simulink model "DCAC"  (R2023b)
settings: Solver=FixedStepDiscrete  StartTime=0.0  StopTime=5  FixedStep=SIM_Ts  RelTol=1e-3
PreLoadFcn:
  | addpath("Sim\");
  | run(Sim_PreLoad_DCAC.mlx);
undefined symbols (not defined in the file): C, f_Vref, L, R_Load, SIM_Ts, t_Vref, Ts, V_DC
libraries: spsSeriesRLCBranchLib x19, spsMosfetLib x12, simulink x10, spsVoltageMeasurementLib x9, spsOnDelayLib x8, spsDCVoltageSourceLib x1, spsGroundLib x1, spsMultimeterLib x1, spspowerguiLib x1
settings Model: Creator=VanillaC  LastModifiedBy=VanillaC
settings DataIOCC: ReturnWorkspaceOutputs=off
settings OptimizationCC: DefaultParameterBehavior=Inlined  EnhancedBackFolding=on  PassReuseOutputArgsAs=Individual arguments  ZeroExternalMemoryAtStartup=off  ZeroInternalMemoryAtStartup=off  OptimizeBlockOrder=speed  DifferentSizesBufferReuse=on  OptimizationCustomize=off  EfficientTunableParamExpr=on
settings DebuggingCC: ParameterTunabilityLossMsg=error
settings SFSimCC: MATLABDynamicMemAlloc=off
settings RTWCC: Description=Embedded Coder  SystemTargetFile=ert.tlc  GenCodeOnly=on  TemplateMakefile=ert_default_tmf
settings CodeAppCC: ForceParamTrailComments=on  IgnoreCustomStorageClasses=off  OperatorAnnotations=on  SimulinkDataObjDesc=on  SFDataObjDesc=on  InsertBlockDesc=on  MATLABSourceComments=on
settings ERTTargetCC: TargetLangStandard=C99 (ISO)  GenerateSampleERTMain=on  SupportContinuousTime=on  InlinedParameterPlacement=NonHierarchical  ERTCustomFileTemplate=example_file_process.tlc

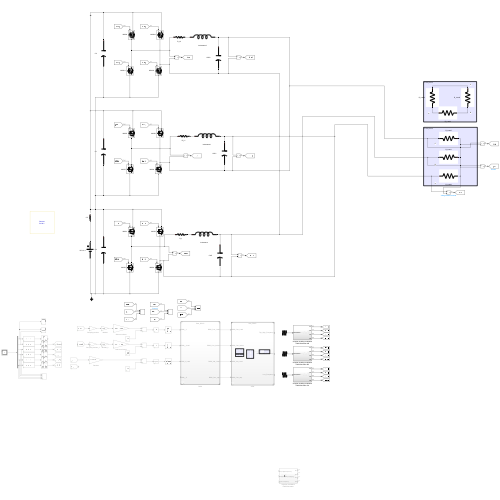
[thumbnail: Simulink's stored preview of the top-level diagram]
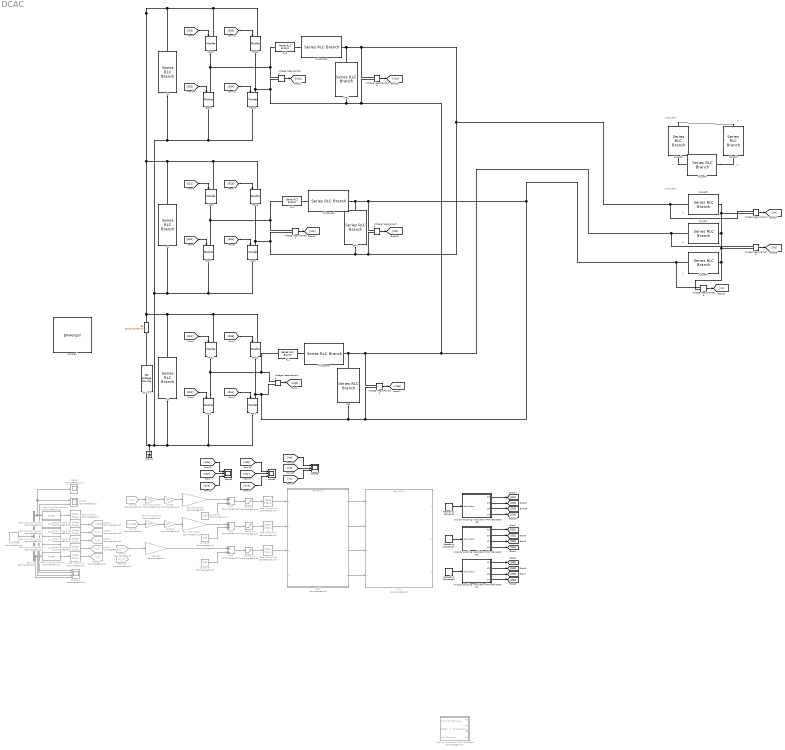
== system DCAC ==
  note: A
  note: Subsystem
  note: B
  note: C
  note: A
  note: Subsystem
  note: C
  note: B
  ASW : ModelReference  Commented=on  ModelNameDialog=Asw_DCAC.slx  SimulationMode=Normal  ModelReferenceVersion=7.2
  Add3 : Sum  Commented=on
  Add4 : Sum  Commented=on
  Add5 : Sum  Commented=on
  BSW : ModelReference  Commented=on  ModelNameDialog=Bsw_DCAC.slx  SimulationMode=Normal  ModelReferenceVersion=1.11
      settings: PortSchema="{\"entries\":[{\"content\":{\"sides\":[{\"content\":{\"connectorIds\":[\"In2\",\"In1\",\"In3\",\"In4\"]},\"type\":\"ConnectorPlacement.EquallySpacedRectSide\",\"uuid\":\"b2b7a57c-7cf1-4c06-9e54-7dc01d62324f\"},{\"content\":{\"connectorIds\":[\"Out1\",\"Out2\",\"Out3\",\"Out4\"],\"side\":\"RIGHT\"},\"type\":\"ConnectorPlacement.EquallySpacedRectSide\",\"uuid\":\"58967db2-deee-4275-8865-8f1f6f5d01b9\"},{\"content\":{\"side\":\"TOP\"},\"type\":\"ConnectorPlacement.EquallySpacedRectSide\",\"uuid\":\"d9088037-5ecd-44ee-9dae-30c0aa6e59e3\"}]},\"type\":\"ConnectorPlacement.EquallySpacedConnector\",\"uuid\":\"be37a7a2-a861-4ca5-b50a-1f8ecf43409b\"}],\"packageUris\":[\"http://schema.mathworks.com/mf0/Connector/R2020b\"],\"version\":\"1.0\"}"
  C1 : spsSeriesRLCBranchLib/Series RLC Branch  LConnTagsString=__new0  RConnTagsString=__new0  BranchType=C  Resistance=1e-9  Inductance=1e-3  SetiL0=off  InitialCurrent=0  Capacitance=2.2e3  Setx0=off  InitialVoltage=0  Measurements=None
  C2 : spsSeriesRLCBranchLib/Series RLC Branch  LConnTagsString=__new0  RConnTagsString=__new0  BranchType=C  Resistance=1e-9  Inductance=1e-3  SetiL0=off  InitialCurrent=0  Capacitance=2.2e3  Setx0=off  InitialVoltage=0  Measurements=None
  C3 : spsSeriesRLCBranchLib/Series RLC Branch  LConnTagsString=__new0  RConnTagsString=__new0  BranchType=C  Resistance=1e-9  Inductance=1e-3  SetiL0=off  InitialCurrent=0  Capacitance=2.2e3  Setx0=off  InitialVoltage=0  Measurements=None
  C5 : spsSeriesRLCBranchLib/Series RLC Branch  LConnTagsString=__new0  RConnTagsString=__new0  BranchType=R  Resistance=1e-10  Inductance=1e-3  SetiL0=off  InitialCurrent=0  Capacitance=2.2e-3  Setx0=off  InitialVoltage=0  Measurements=None
  CAP : spsSeriesRLCBranchLib/Series RLC Branch  LConnTagsString=__new0  RConnTagsString=__new0  BranchType=C  Resistance=1000  Inductance=1e-3  SetiL0=off  InitialCurrent=0  Capacitance=C  Setx0=off  InitialVoltage=0  Measurements=Branch voltage and current
  CAP1 : spsSeriesRLCBranchLib/Series RLC Branch  LConnTagsString=__new0  RConnTagsString=__new0  BranchType=C  Resistance=1000  Inductance=1e-3  SetiL0=off  InitialCurrent=0  Capacitance=C  Setx0=off  InitialVoltage=0  Measurements=Branch voltage and current
  CAP2 : spsSeriesRLCBranchLib/Series RLC Branch  LConnTagsString=__new0  RConnTagsString=__new0  BranchType=C  Resistance=1000  Inductance=1e-3  SetiL0=off  InitialCurrent=0  Capacitance=C  Setx0=off  InitialVoltage=0  Measurements=Branch voltage and current
  Constant3 : Constant  Commented=on  Value=1.65  OutDataTypeStr=single  SampleTime=-1
  Constant4 : Constant  Commented=on  Value=1.65  OutDataTypeStr=single  SampleTime=-1
  Constant5 : Constant  Commented=on  Value=1.65  OutDataTypeStr=single  SampleTime=-1
  DC Vin 1 : spsDCVoltageSourceLib/DC Voltage Source  Amplitude=V_DC  Measurements=None
  Data Type Conversion{1..6} (6 alike) : DataTypeConversion  Commented=on  OutDataTypeStr=single  SaturateOnIntegerOverflow=off  RndMeth=Floor
  Demux1 : Demux  Commented=on  Outputs=6
  From16 : From  Commented=on  GotoTag=U_C
  From19 : From  Commented=on  GotoTag=I_Load
  From20 : From  Commented=on  GotoTag=I_L
  From21 : From  Commented=on  GotoTag=U_Load
  Gain error factor : Gain  Commented=on  Gain=3000/(10+3000)
  Gain error factor1 : Gain  Commented=on  Gain=3000/(10+3000)
  Goto19 : Goto  Commented=on  GotoTag=I_Load
  Goto20 : Goto  Commented=on  GotoTag=U_L
  Goto21 : Goto  Commented=on  GotoTag=I_L
  Goto22 : Goto  Commented=on  GotoTag=U_C
  Goto23 : Goto  Commented=on  GotoTag=I_C
  Ground : spsGroundLib/Ground  LConnTagsString=a
  INA296 : Gain  Commented=on  Gain=100
  INA296_2 : Gain  Commented=on  Gain=100
  Inductance : spsSeriesRLCBranchLib/Series RLC Branch  LConnTagsString=__new0  RConnTagsString=__new0  BranchType=L  Resistance=0.005  Inductance=L  SetiL0=off  InitialCurrent=0  Capacitance=470e-6  Setx0=off  InitialVoltage=0  Measurements=Branch voltage and current
  Inductance1 : spsSeriesRLCBranchLib/Series RLC Branch  LConnTagsString=__new0  RConnTagsString=__new0  BranchType=L  Resistance=0.005  Inductance=L  SetiL0=off  InitialCurrent=0  Capacitance=470e-6  Setx0=off  InitialVoltage=0  Measurements=Branch voltage and current
  Inductance2 : spsSeriesRLCBranchLib/Series RLC Branch  LConnTagsString=__new0  RConnTagsString=__new0  BranchType=L  Resistance=0.005  Inductance=L  SetiL0=off  InitialCurrent=0  Capacitance=470e-6  Setx0=off  InitialVoltage=0  Measurements=Branch voltage and current
  MOS{1..12} (12 alike) : spsMosfetLib/Mosfet  Ron=1e-9  Lon=0  Rd=1e-9  Vfd=0.7  IC=0  Rs=1e5  Cs=inf  Measurements=off
  Multimeter : spsMultimeterLib/Multimeter  Commented=on  L=8  sel=[4 8 2 6 1 5]  yselected={}  Gain=[1 1 1 1 1 1]  OutputType=Complex  PlotAtSimulationStop=off  PhasorSimulation=off
  R_L : spsSeriesRLCBranchLib/Series RLC Branch  LConnTagsString=__new0  RConnTagsString=__new0  BranchType=R  Resistance=1e-10  Inductance=1e-3  SetiL0=off  InitialCurrent=0  Capacitance=470e-6  Setx0=off  InitialVoltage=0  Measurements=None
  R_L1 : spsSeriesRLCBranchLib/Series RLC Branch  LConnTagsString=__new0  RConnTagsString=__new0  BranchType=R  Resistance=1e-10  Inductance=1e-3  SetiL0=off  InitialCurrent=0  Capacitance=470e-6  Setx0=off  InitialVoltage=0  Measurements=None
  R_L2 : spsSeriesRLCBranchLib/Series RLC Branch  LConnTagsString=__new0  RConnTagsString=__new0  BranchType=R  Resistance=1e-10  Inductance=1e-3  SetiL0=off  InitialCurrent=0  Capacitance=470e-6  Setx0=off  InitialVoltage=0  Measurements=None
  R_Load{1..6} (6 alike) : spsSeriesRLCBranchLib/Series RLC Branch  LConnTagsString=__new0  RConnTagsString=__new0  BranchType=R  Resistance=R_Load  Inductance=1e-3  SetiL0=off  InitialCurrent=0  Capacitance=470e-6  Setx0=off  InitialVoltage=0  Measurements=Branch voltage and current
  Rate Transition{,1..8} (9 alike) : RateTransition  Commented=on  OutPortSampleTime=Ts
  Repeating Sequence : simulink/Sources/Repeating Sequence  rep_seq_t=[0 4e-3 (t_Vref/3)-(8e-3) t_Vref/3 t_Vref/3+4e-3 (t_Vref*2/3)-(8e-3) (t_Vref*2/3) (t_Vref*3/3)]  rep_seq_y=[0 -0.3 -0.3 0 0.3 0.3 0 0]
  Repeating Sequence1 : simulink/Sources/Repeating Sequence  rep_seq_t=[0 t_Vref/3 (t_Vref/3)+(4e-3) (t_Vref*2/3)-(8e-3) (t_Vref*2/3) (t_Vref*2/3)+(4e-3) (t_Vref*3/3)-(8e-3) (t_Vref*3/3)]  rep_seq_y=[0 0 -0.3 -0.3 0 0.3 0.3 0]
  Repeating Sequence2 : simulink/Sources/Repeating Sequence  rep_seq_t="[0 4e-3 (t_Vref/3)-(8e-3) t_Vref/3  t_Vref*2/3 t_Vref*2/3+(4e-3)  t_Vref*3/3-(8e-3)  t_Vref*3/3  ]"  rep_seq_y=[0 0.3 0.3 0 0 -0.3 -0.3 0]
  Resister : Gain  Commented=on  Gain=(15)/(470+15)
  Sampling resistor : Gain  Commented=on  Gain=0.015
  Sampling resistor_2 : Gain  Commented=on  Gain=0.015
  Saturation : Saturate  Commented=on  UpperLimit=3.3  LowerLimit=0
  Saturation1 : Saturate  Commented=on  UpperLimit=3.3  LowerLimit=0
  Saturation2 : Saturate  Commented=on  UpperLimit=3.3  LowerLimit=0
  Scope1 : Scope  Commented=on
  Scope11 : Scope  Commented=on  NumInputPorts=4
  Scope2 : Scope  NumInputPorts=3
  Scope3 : Scope  NumInputPorts=3
  Scope5 : Scope  NumInputPorts=3
  Scope6 : Scope  Commented=on  NumInputPorts=2
  Unipolar doubling modulation PWM Generator AB : Subsystem
  Unipolar doubling modulation PWM Generator BC : Subsystem
  Unipolar doubling modulation PWM Generator CA : Subsystem
  Unipolar modulation PWM Generator : Subsystem  Commented=on
  Voltage Measurement{1..9} (9 alike) : spsVoltageMeasurementLib/Voltage Measurement  PhasorSimulation=off  OutputType=Complex  PSBequivalent=0
  powergui : spspowerguiLib/powergui  Priority=1  SimulationMode=Discrete  SampleTime=SIM_Ts  frequency=60  Iterations=50  frequencyindice=0  Pbase=100e6  ErrMax=1e-4  UnitsV=kV  UnitsW=MW  buscounter=0  FunctionMessages=off  echomessages=off  EnableUseOfTLC=off  CurrentSourceSwitches=off  DisableSnubberDevices=off  DisableRonSwitches=off  DisableVfSwitches=off  DisplayEquations=off  AutomaticDiscreteSolvers=off  SolverType=Tustin/Backward Euler (TBE)  Interpol=off  ExternalGateDelay=off  methode=off  Ts=100  x0status=blocks  SPID=on  SwTol=0  HookPort=off  NonlinearTolerance=1e-4  nMaxIteration=100  ContinueOnMaxIteration=off  RestoreLinks=warning  ResistiveCurrentMeasurement=off  Frange=[0:2:500]  Ylog=off  Xlog=on  ShowGrid=off  save=off  variable=ZData  structure=0  ZoomFFT=off  StartTime=0.0  cycles=1  DisplayStyle=1  fundamental=60  FreqAxis=off  MaxFrequency=1000  frequencyindicesteady=1  RmsSteady=1  display=off
  wires:
  [G13] -> MOS2/1
  [G14] -> MOS4/1
  [G12] -> MOS3/1
  [G11] -> MOS1/1
  Voltage Measurement1/1 -> [Uab]
  Multimeter/1 -> Demux1/1
  Demux1/1 -> Scope6/1, Scope1/1, Data Type Conversion1/1
  Demux1/2 -> Scope6/2, Data Type Conversion2/1
  Demux1/3 -> Scope11/1, Data Type Conversion4/1
  Demux1/4 -> Scope11/2, Data Type Conversion3/1
  Data Type Conversion1/1 -> Rate Transition/1
  Data Type Conversion2/1 -> Rate Transition1/1
  Data Type Conversion3/1 -> Rate Transition3/1
  Data Type Conversion4/1 -> Rate Transition2/1
  Rate Transition1/1 -> Goto19/1
  Rate Transition2/1 -> Goto20/1
  Rate Transition3/1 -> Goto21/1
  Rate Transition4/1 -> Goto22/1
  Data Type Conversion5/1 -> Rate Transition4/1
  Data Type Conversion6/1 -> Rate Transition5/1
  Rate Transition5/1 -> Goto23/1
  Demux1/5 -> Scope11/3, Data Type Conversion5/1
  From20/1 -> Sampling resistor/1
  Demux1/6 -> Scope11/4, Data Type Conversion6/1
  From19/1 -> Sampling resistor_2/1
  Sampling resistor/1 -> INA296/1
  Sampling resistor_2/1 -> INA296_2/1
  Add3/1 -> Saturation/1
  Constant3/1 -> Add3/2
  Gain error factor/1 -> Add3/1
  INA296/1 -> Gain error factor/1
  Add4/1 -> Saturation1/1
  Constant4/1 -> Add4/2
  Gain error factor1/1 -> Add4/1
  INA296_2/1 -> Gain error factor1/1
  Saturation/1 -> Rate Transition6/1
  Saturation1/1 -> Rate Transition7/1
  Constant5/1 -> Add5/2
  Resister/1 -> Add5/1
  Add5/1 -> Saturation2/1
  Rate Transition6/1 -> BSW/2
  Rate Transition7/1 -> BSW/1
  Rate Transition8/1 -> BSW/3
  BSW/1 -> ASW/1
  BSW/2 -> ASW/2
  BSW/3 -> ASW/3
  BSW/4 -> ASW/4
  Saturation2/1 -> Rate Transition8/1
  [Uab] -> Scope5/1
  From21/1 -> Resister/1
  Voltage Measurement5/1 -> [Vab]
  [G22] -> MOS7/1
  [G21] -> MOS5/1
  [G23] -> MOS6/1
  [G24] -> MOS8/1
  [G32] -> MOS11/1
  [G31] -> MOS9/1
  [G33] -> MOS10/1
  [G34] -> MOS12/1
  Unipolar doubling modulation PWM Generator AB/1(G1) -> [G11]
  Unipolar doubling modulation PWM Generator AB/2(G2) -> [G12]
  Unipolar doubling modulation PWM Generator AB/3(G3) -> [G13]
  Unipolar doubling modulation PWM Generator AB/4(G4) -> [G14]
  Unipolar doubling modulation PWM Generator BC/4(G4) -> [G24]
  Unipolar doubling modulation PWM Generator BC/2(G2) -> [G22]
  Unipolar doubling modulation PWM Generator BC/1(G1) -> [G21]
  Unipolar doubling modulation PWM Generator BC/3(G3) -> [G23]
  Unipolar doubling modulation PWM Generator CA/4(G4) -> [G34]
  Unipolar doubling modulation PWM Generator CA/2(G2) -> [G32]
  Unipolar doubling modulation PWM Generator CA/1(G1) -> [G31]
  Unipolar doubling modulation PWM Generator CA/3(G3) -> [G33]
  Voltage Measurement2/1 -> [Ubc]
  [Ubc] -> Scope5/2
  Voltage Measurement3/1 -> [Uca]
  [Uca] -> Scope5/3
  Voltage Measurement4/1 -> [Vbc]
  Voltage Measurement6/1 -> [Vca]
  [Vbc] -> Scope2/2
  [Vab] -> Scope2/1
  [Vca] -> Scope2/3
  Voltage Measurement7/1 -> [Va]
  Voltage Measurement8/1 -> [Vb]
  Voltage Measurement9/1 -> [Vc]
  [Vb] -> Scope3/2
  [Va] -> Scope3/1
  [Vc] -> Scope3/3
  Repeating Sequence/1 -> Unipolar doubling modulation PWM Generator AB/1(Modulation)
  Repeating Sequence1/1 -> Unipolar doubling modulation PWM Generator BC/1(Modulation)
  Repeating Sequence2/1 -> Unipolar doubling modulation PWM Generator CA/1(Modulation)
  connections:
  MOS3/LConn1 -- Voltage Measurement1/LConn1 -- R_L/LConn1 -- MOS1/RConn1
  DC Vin 1/RConn1 -- C5/RConn1
  MOS11/RConn1 -- MOS12/RConn1 -- C2/RConn1 -- DC Vin 1/LConn1 -- Ground/LConn1 -- C3/RConn1 -- MOS4/RConn1 -- MOS3/RConn1 -- C1/RConn1 -- MOS8/RConn1 -- MOS7/RConn1
  R_L/RConn1 -- Inductance/LConn1
  MOS12/LConn1 -- MOS10/RConn1 -- Voltage Measurement3/LConn2 -- Voltage Measurement6/LConn2 -- R_Load1/RConn1 -- Voltage Measurement8/LConn1 -- CAP/LConn1 -- Inductance/RConn1 -- Voltage Measurement5/LConn1 -- CAP2/RConn1
  C3/LConn1 -- C5/LConn1 -- C2/LConn1 -- MOS9/LConn1 -- MOS10/LConn1 -- C1/LConn1 -- MOS5/LConn1 -- MOS6/LConn1 -- MOS1/LConn1 -- MOS2/LConn1
  MOS8/LConn1 -- Voltage Measurement4/LConn2 -- Voltage Measurement6/LConn1 -- CAP2/LConn1 -- Inductance2/RConn1 -- Voltage Measurement7/LConn1 -- R_Load5/RConn1 -- CAP1/RConn1 -- Voltage Measurement2/LConn2 -- MOS6/RConn1
  Inductance1/RConn1 -- Voltage Measurement4/LConn1 -- MOS2/RConn1 -- MOS4/LConn1 -- Voltage Measurement1/LConn2 -- CAP/RConn1 -- Voltage Measurement5/LConn2 -- Voltage Measurement9/LConn1 -- R_Load6/LConn1 -- CAP1/LConn1
  Voltage Measurement2/LConn1 -- R_L1/LConn1 -- MOS7/LConn1 -- MOS5/RConn1
  R_L1/RConn1 -- Inductance1/LConn1
  Voltage Measurement3/LConn1 -- R_L2/LConn1 -- MOS11/LConn1 -- MOS9/RConn1
  R_L2/RConn1 -- Inductance2/LConn1
  R_Load5/LConn1 -- Voltage Measurement7/LConn2 -- R_Load1/LConn1 -- Voltage Measurement8/LConn2 -- Voltage Measurement9/LConn2 -- R_Load6/RConn1
  R_Load4/RConn1 -- R_Load3/RConn1
  R_Load2/LConn1 -- R_Load3/LConn1
  R_Load2/RConn1 -- R_Load4/LConn1

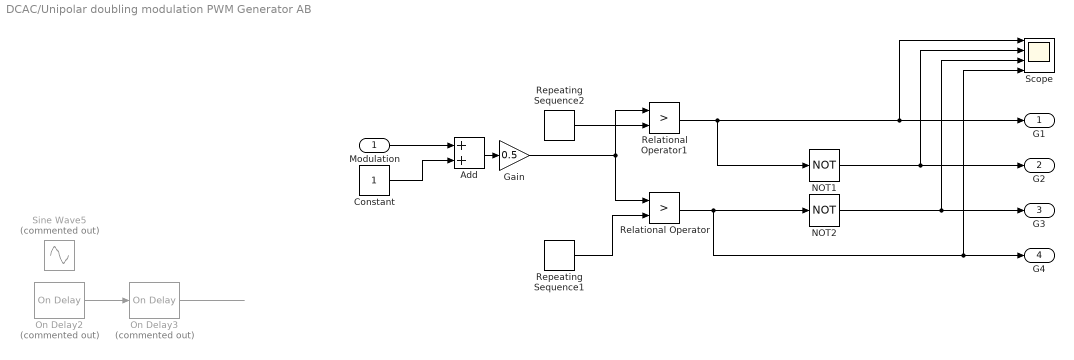
== system DCAC/Unipolar doubling modulation PWM Generator AB ==
  Modulation : Inport
  Add : Sum
  Constant : Constant
  Gain : Gain  Gain=0.5
  NOT1 : Logic  Operator=NOT  IconShape=distinctive  AllPortsSameDT=off  OutDataTypeStr=boolean
  NOT2 : Logic  Operator=NOT  IconShape=distinctive  AllPortsSameDT=off  OutDataTypeStr=boolean
  On Delay2 : spsOnDelayLib/On Delay  Commented=on  DelayType=On delay  delay=10e-9  ic=0  Ts=0
  On Delay3 : spsOnDelayLib/On Delay  Commented=on  DelayType=Off delay  delay=10e-9  ic=0  Ts=0
  Relational Operator : RelationalOperator  Operator=>  OutDataTypeStr=boolean  RndMeth=Simplest  InputSameDT=off
  Relational Operator1 : RelationalOperator  Operator=>  OutDataTypeStr=boolean  RndMeth=Simplest  InputSameDT=off
  Repeating Sequence1 : simulink/Sources/Repeating Sequence  rep_seq_t=[0 Ts/2 Ts]  rep_seq_y=[0 1 0]
  Repeating Sequence2 : simulink/Sources/Repeating Sequence  rep_seq_t=[0 Ts/2 Ts]  rep_seq_y=[1 0 1]
  Scope : Scope  NumInputPorts=4
  Sine Wave5 : Sin  Commented=on  Frequency=f_Vref  SampleTime=Ts
  G1 : Outport
  G2 : Outport  Port=2
  G3 : Outport  Port=3
  G4 : Outport  Port=4
  wires:
  Constant/1 -> Add/2
  Add/1 -> Gain/1
  On Delay3/1 -> ?
  On Delay2/1 -> On Delay3/1
  ? -> On Delay2/1
  Repeating Sequence2/1 -> Relational Operator1/2
  Repeating Sequence1/1 -> Relational Operator/2
  Gain/1 -> Relational Operator/1, Relational Operator1/1
  Relational Operator1/1 -> NOT1/1, Scope/1, G1/1
  NOT1/1 -> Scope/2, G2/1
  NOT2/1 -> Scope/3, G3/1
  Relational Operator/1 -> Scope/4, G4/1, NOT2/1
  Modulation/1 -> Add/1

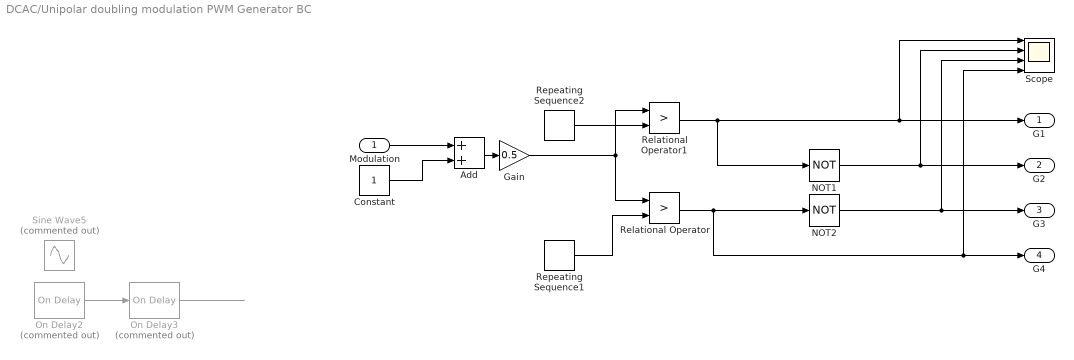
== system DCAC/Unipolar doubling modulation PWM Generator BC ==
  Modulation : Inport
  Add : Sum
  Constant : Constant
  Gain : Gain  Gain=0.5
  NOT1 : Logic  Operator=NOT  IconShape=distinctive  AllPortsSameDT=off  OutDataTypeStr=boolean
  NOT2 : Logic  Operator=NOT  IconShape=distinctive  AllPortsSameDT=off  OutDataTypeStr=boolean
  On Delay2 : spsOnDelayLib/On Delay  Commented=on  DelayType=On delay  delay=10e-9  ic=0  Ts=0
  On Delay3 : spsOnDelayLib/On Delay  Commented=on  DelayType=Off delay  delay=10e-9  ic=0  Ts=0
  Relational Operator : RelationalOperator  Operator=>  OutDataTypeStr=boolean  RndMeth=Simplest  InputSameDT=off
  Relational Operator1 : RelationalOperator  Operator=>  OutDataTypeStr=boolean  RndMeth=Simplest  InputSameDT=off
  Repeating Sequence1 : simulink/Sources/Repeating Sequence  rep_seq_t=[0 Ts/2 Ts]  rep_seq_y=[0 1 0]
  Repeating Sequence2 : simulink/Sources/Repeating Sequence  rep_seq_t=[0 Ts/2 Ts]  rep_seq_y=[1 0 1]
  Scope : Scope  NumInputPorts=4
  Sine Wave5 : Sin  Commented=on  Frequency=f_Vref  SampleTime=Ts
  G1 : Outport
  G2 : Outport  Port=2
  G3 : Outport  Port=3
  G4 : Outport  Port=4
  wires:
  Constant/1 -> Add/2
  Add/1 -> Gain/1
  On Delay3/1 -> ?
  On Delay2/1 -> On Delay3/1
  ? -> On Delay2/1
  Repeating Sequence2/1 -> Relational Operator1/2
  Repeating Sequence1/1 -> Relational Operator/2
  Gain/1 -> Relational Operator/1, Relational Operator1/1
  Relational Operator1/1 -> NOT1/1, Scope/1, G1/1
  NOT1/1 -> Scope/2, G2/1
  NOT2/1 -> Scope/3, G3/1
  Relational Operator/1 -> Scope/4, G4/1, NOT2/1
  Modulation/1 -> Add/1

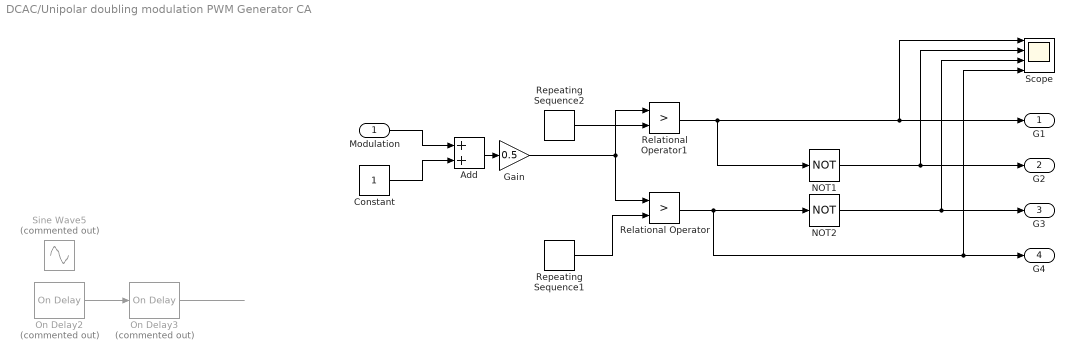
== system DCAC/Unipolar doubling modulation PWM Generator CA ==
  Modulation : Inport
  Add : Sum
  Constant : Constant
  Gain : Gain  Gain=0.5
  NOT1 : Logic  Operator=NOT  IconShape=distinctive  AllPortsSameDT=off  OutDataTypeStr=boolean
  NOT2 : Logic  Operator=NOT  IconShape=distinctive  AllPortsSameDT=off  OutDataTypeStr=boolean
  On Delay2 : spsOnDelayLib/On Delay  Commented=on  DelayType=On delay  delay=10e-9  ic=0  Ts=0
  On Delay3 : spsOnDelayLib/On Delay  Commented=on  DelayType=Off delay  delay=10e-9  ic=0  Ts=0
  Relational Operator : RelationalOperator  Operator=>  OutDataTypeStr=boolean  RndMeth=Simplest  InputSameDT=off
  Relational Operator1 : RelationalOperator  Operator=>  OutDataTypeStr=boolean  RndMeth=Simplest  InputSameDT=off
  Repeating Sequence1 : simulink/Sources/Repeating Sequence  rep_seq_t=[0 Ts/2 Ts]  rep_seq_y=[0 1 0]
  Repeating Sequence2 : simulink/Sources/Repeating Sequence  rep_seq_t=[0 Ts/2 Ts]  rep_seq_y=[1 0 1]
  Scope : Scope  NumInputPorts=4
  Sine Wave5 : Sin  Commented=on  Frequency=f_Vref  SampleTime=Ts
  G1 : Outport
  G2 : Outport  Port=2
  G3 : Outport  Port=3
  G4 : Outport  Port=4
  wires:
  Constant/1 -> Add/2
  Add/1 -> Gain/1
  On Delay3/1 -> ?
  On Delay2/1 -> On Delay3/1
  ? -> On Delay2/1
  Repeating Sequence2/1 -> Relational Operator1/2
  Repeating Sequence1/1 -> Relational Operator/2
  Gain/1 -> Relational Operator/1, Relational Operator1/1
  Relational Operator1/1 -> NOT1/1, Scope/1, G1/1
  NOT1/1 -> Scope/2, G2/1
  NOT2/1 -> Scope/3, G3/1
  Relational Operator/1 -> Scope/4, G4/1, NOT2/1
  Modulation/1 -> Add/1

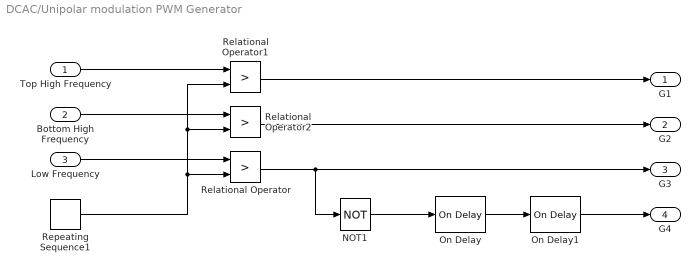
== system DCAC/Unipolar modulation PWM Generator ==
  Top High Frequency : Inport
  Bottom High Frequency : Inport  Port=2
  Low Frequency : Inport  Port=3
  NOT1 : Logic  Operator=NOT  IconShape=distinctive  AllPortsSameDT=off  OutDataTypeStr=boolean
  On Delay : spsOnDelayLib/On Delay  DelayType=On delay  delay=10e-9  ic=0  Ts=0
  On Delay1 : spsOnDelayLib/On Delay  DelayType=Off delay  delay=10e-9  ic=0  Ts=0
  Relational Operator : RelationalOperator  Operator=>  OutDataTypeStr=boolean  RndMeth=Simplest  InputSameDT=off
  Relational Operator1 : RelationalOperator  Operator=>  OutDataTypeStr=boolean  RndMeth=Simplest  InputSameDT=off
  Relational Operator2 : RelationalOperator  Operator=>  OutDataTypeStr=boolean  RndMeth=Simplest  InputSameDT=off
  Repeating Sequence1 : simulink/Sources/Repeating Sequence  rep_seq_t=[0 Ts/2 Ts]  rep_seq_y=[0 1 0]
  G1 : Outport
  G2 : Outport  Port=2
  G3 : Outport  Port=3
  G4 : Outport  Port=4
  wires:
  Repeating Sequence1/1 -> Relational Operator/2, Relational Operator2/2, Relational Operator1/2
  NOT1/1 -> On Delay/1
  Relational Operator/1 -> G3/1, NOT1/1
  Relational Operator1/1 -> G1/1
  Top High Frequency/1 -> Relational Operator1/1
  Relational Operator2/1 -> G2/1
  Bottom High Frequency/1 -> Relational Operator2/1
  Low Frequency/1 -> Relational Operator/1
  On Delay/1 -> On Delay1/1
  On Delay1/1 -> G4/1
